simulink model "CranePIDv01"  (R2016b)
settings: Solver=ode45  StartTime=0.0  StopTime=280  RelTol=1e-3  EnableMultiTasking=on
PostLoadFcn:
  | plot_timeseries(Simulation_results);
undefined symbols (not defined in the file): A, adinchannels, adinchannelsencoders, adingain, adingainencoders, adinoffs, adinoffsencoders, B, C, D, daoutchannels, daoutgain, daoutoffs, h, Humusoft, MF634, sigbuilder_block
libraries: sldrtlib x3, simulink x3, dspsrcs4 x1
settings Model: Creator=rbabuska  LastModifiedBy=tcbooij
settings DataIOCC: LimitDataPoints=on  SaveFormat=Array
settings OptimizationCC: ExpressionDepthLimit=2147483647  LifeSpan=inf
settings DebuggingCC: AllowSymbolicDim=off  StateNameClashWarn=warning  SFUnexpectedBacktrackingDiag=warning  SFNoUnconditionalDefaultTransitionDiag=warning  SFExecutionAtInitializationDiag=none
settings HardwareCC: ProdBitPerPointer=32  ProdBitPerSizeT=32  ProdBitPerPtrDiffT=32  ProdLargestAtomicFloat=None  ProdIntDivRoundTo=Undefined  ProdEndianess=Unspecified  ProdWordSize=32  ProdHWDeviceType=32-bit Generic
settings ModelReferenceCC: PropagateSignalLabelsOutOfModel=off
settings GRTTargetCC: TargetLangStandard=C89/C90 (ANSI)  GeneratePreprocessorConditionals=Disable all  CombineOutputUpdateFcns=off  GRTInterface=on
settings ConfigComp: CovMetricSettings=dw  CovHtmlReporting=on  CovSaveCumulativeToWorkspaceVar=on  CovSaveSingleToWorkspaceVar=on  CovExternalEMLEnable=off

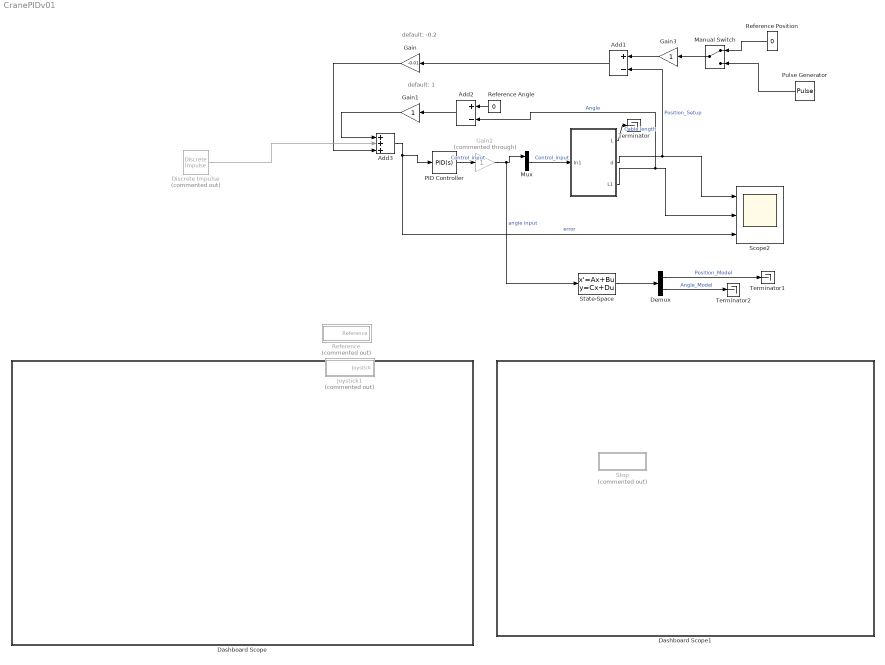
== system CranePIDv01 ==
  note: default: -0.2
  note: default: 1
  " Reference Angle" : Constant  Value=0
  " " : Subsystem  LoadFcn=hwinit  InitFcn=hwinit  mask{h=h}
      mask prompts: h "Sampling period [s]"
      mask Display: disp('Crane')
  Add1 : Sum  Inputs=+-
  Add2 : Sum  Inputs=+-
  Add3 : Sum  Inputs=3
  Dashboard Scope : Subsystem  DialogController=hmiCreateDDGDialog  IsWebBlock=on  mask(MWDashboardBlock){webBlockId=2a6f5fa7-1f9e-4fe4-9305-f01df55b8dfe, webBlockType=sdiscope, ShowInitialText=on, HMISrcModelName=CranePIDv01}
      mask prompts: webBlockId "WebBlock Id"; webBlockType "WebBlock Type"; HMISrcModelName "Source Model"
      mask help: SimulinkHMI:dialogs:HMIScopeDialogDesc
      mask Help: helpview([docroot '/mapfiles/simulink.map'], 'hmi_scope')
      mask Display:
      | if strcmp(get_param(bdroot(gcb),'BlockDiagramType'), 'library')
      |     image([(matlabroot) '/toolbox/simulink/hmi/icons/DashboardScope.png']);
      | end
  Dashboard Scope1 : Subsystem  DialogController=hmiCreateDDGDialog  IsWebBlock=on  mask(MWDashboardBlock){webBlockId=26260313-c547-41b7-b078-74ae54bbf42b, webBlockType=sdiscope, ShowInitialText=on, HMISrcModelName=CranePIDv01}
      mask prompts: webBlockId "WebBlock Id"; webBlockType "WebBlock Type"; HMISrcModelName "Source Model"
      mask help: SimulinkHMI:dialogs:HMIScopeDialogDesc
      mask Help: helpview([docroot '/mapfiles/simulink.map'], 'hmi_scope')
      mask Display:
      | if strcmp(get_param(bdroot(gcb),'BlockDiagramType'), 'library')
      |     image([(matlabroot) '/toolbox/simulink/hmi/icons/DashboardScope.png']);
      | end
  Demux : Demux  Outputs=2
  Discrete Impulse : dspsrcs4/Discrete  Impulse  Commented=on  Delay=0  SampleTime=1  FrameSample=1  OutputFrames=off  dataType=double  isSigned=on  wordLen=16  udDataType=sfix(16)  fracBitsMode=Best precision  numFracBits=15  OutDataTypeStr=double  LastOutDataTypeStr=double
  Gain : Gain  Gain=-0.01
  Gain1 : Gain
  Gain2 : Gain  Commented=through
  Gain3 : Gain
  Joystick1 : Subsystem  Commented=on
      mask Display: disp('Joystick')
  Manual Switch : ManualSwitch
  Mux : Mux  Inputs=2
  PID Controller : simulink/Continuous/PID Controller  Controller=PID  TimeDomain=Continuous-time  SampleTime=-1  IntegratorMethod=Forward Euler  FilterMethod=Forward Euler  Form=Parallel  UseFilter=on  ControllerParametersSource=internal  P=15  I=1  D=2  N=1  InitialConditionSource=internal  InitialConditionForIntegrator=0  InitialConditionForFilter=0  ExternalReset=none  LimitOutput=off  UpperSaturationLimit=inf  LowerSaturationLimit=-inf  LinearizeAsGain=on  AntiWindupMode=none  Kb=1  TrackingMode=off  Kt=1  PParamMin=[]  PParamMax=[]  IParamMin=[]  IParamMax=[]  DParamMin=[]  DParamMax=[]  NParamMin=[]  NParamMax=[]  KbParamMin=[]  KbParamMax=[]  KtParamMin=[]  KtParamMax=[]  POutMin=[]  POutMax=[]  IOutMin=[]  IOutMax=[]  DOutMin=[]  DOutMax=[]  NOutMin=[]  NOutMax=[]  KbOutMin=[]  KbOutMax=[]  KtOutMin=[]  KtOutMax=[]  IntegratorOutMin=[]  IntegratorOutMax=[]  FilterOutMin=[]  FilterOutMax=[]  SumOutMin=[]  SumOutMax=[]  SumI1OutMin=[]  SumI1OutMax=[]  SumI2OutMin=[]  SumI2OutMax=[]  SumI3OutMin=[]  SumI3OutMax=[]  SumDOutMin=[]  SumDOutMax=[]  SaturationOutMin=[]  SaturationOutMax=[]  IntegratorContinuousStateAttributes=''  IntegratorStateMustResolveToSignalObject=off  IntegratorRTWStateStorageClass=Auto  FilterContinuousStateAttributes=''  FilterStateMustResolveToSignalObject=off  FilterRTWStateStorageClass=Auto  DifferentiatorICPrevScaledInput=0  DifferentiatorOutMin=[]  DifferentiatorOutMax=[]
  Pulse Generator : DiscretePulseGenerator  PulseType=Time based  Amplitude=15  Period=20  PulseWidth=50  PhaseDelay=2
  Reference : Subsystem  Commented=on
      mask Display: disp('Reference')
  Reference Position : Constant  Value=0
  Scope2 : Scope  NumInputPorts=3
  State-Space : StateSpace  A=A  B=B  C=C  D=D  X0=0
  Stop : Subsystem  Commented=on
      mask Display: disp('Stop')
  Terminator : Terminator
  Terminator1 : Terminator
  Terminator2 : Terminator
  wires:
  " "/3(L1) -> Add2/2, Scope2/2  "Angle"
  " "/2(d) -> Add1/2, Scope2/1  "Position_Setup"
  Add3/1 -> PID Controller/1, Scope2/3  "error"
  " Reference Angle"/1 -> Add2/1
  Add2/1 -> Gain1/1
  Add1/1 -> Gain/1
  Gain/1 -> Add3/3
  Discrete Impulse/1 -> Add3/2
  Gain1/1 -> Add3/1
  " "/1(L) -> Terminator/1  "Cable length"
  PID Controller/1 -> Gain2/1  "Control_input"
  Mux/1 -> " "/1(In1)  "Control_input"
  Gain2/1 -> State-Space/1, Mux/1  "angle input"
  Gain3/1 -> Add1/1
  Reference Position/1 -> Manual Switch/1
  State-Space/1 -> Demux/1
  Demux/2 -> Terminator2/1  "Angle_Model"
  Demux/1 -> Terminator1/1  "Position_Model"
  Manual Switch/1 -> Gain3/1
  Pulse Generator/1 -> Manual Switch/2

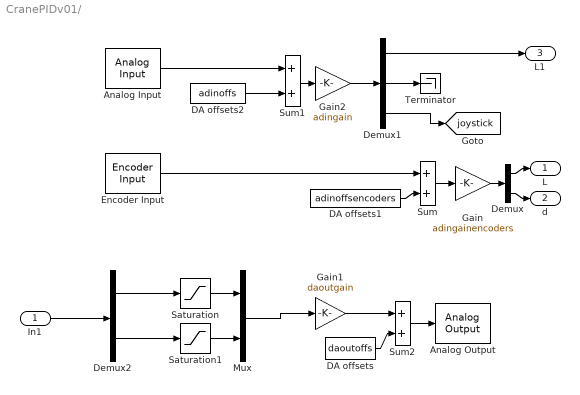
== system CranePIDv01/  ==
  In1 : Inport
  Analog Input : sldrtlib/Analog Input  SampleTime=h  MaxMissedTicks=ticklost  ShowMissedTicks=off  YieldWhenWaiting=off  DrvName=Humusoft/MF634  DrvAddress=4294967295  DrvOptions=0  Channels=[adinchannels]  RangeMode=2  VoltRange=1  DataType=1
      settings: AttributesFormatString=Humusoft\nMF634 [auto]
  Analog Output : sldrtlib/Analog Output  SampleTime=h  MaxMissedTicks=ticklost  ShowMissedTicks=off  YieldWhenWaiting=off  DrvName=Humusoft/MF634  DrvAddress=4294967295  DrvOptions=0  Channels=[daoutchannels]  RangeMode=2  VoltRange=1  InitialValue=0  FinalValue=0
      settings: AttributesFormatString=Humusoft\nMF634 [auto]
  DA offsets : Constant  Value=daoutoffs
  DA offsets1 : Constant  Value=adinoffsencoders
  DA offsets2 : Constant  Value=adinoffs
  Demux : Demux  Outputs=2
  Demux1 : Demux  Outputs=[1 1 2]
  Demux2 : Demux  Outputs=2
  Encoder Input : sldrtlib/Encoder Input  SampleTime=h  MaxMissedTicks=ticklost  ShowMissedTicks=off  YieldWhenWaiting=off  DrvName=Humusoft/MF634  DrvAddress=4294967295  DrvOptions=0  Channels=[adinchannelsencoders]  QuadMode=3  IndexPulse=1  InputFilter=Inf  DataType=1
      settings: AttributesFormatString=Humusoft\nMF634 [auto]
  Gain : Gain  Gain=adingainencoders  SaturateOnIntegerOverflow=on  OutDataTypeStr=Inherit: Same as input  ParamDataTypeStr=Inherit: Same as input
  Gain1 : Gain  Gain=daoutgain  SaturateOnIntegerOverflow=on  OutDataTypeStr=Inherit: Same as input  ParamDataTypeStr=Inherit: Same as input
  Gain2 : Gain  Gain=adingain  SaturateOnIntegerOverflow=on  OutDataTypeStr=Inherit: Same as input  ParamDataTypeStr=Inherit: Same as input
  Mux : Mux  Inputs=2
  Saturation : Saturate  UpperLimit=10  LowerLimit=-10
  Saturation1 : Saturate  UpperLimit=10  LowerLimit=-10
  Sum : Sum  SaturateOnIntegerOverflow=on  InputSameDT=on  OutDataTypeStr=Inherit: Same as first input
  Sum1 : Sum  SaturateOnIntegerOverflow=on  InputSameDT=on  OutDataTypeStr=Inherit: Same as first input
  Sum2 : Sum  SaturateOnIntegerOverflow=on  InputSameDT=on  OutDataTypeStr=Inherit: Same as first input
  Terminator : Terminator
  L : Outport  Tag=Position
  d : Outport  Tag=Cable length  Port=2
  L1 : Outport  Tag=Position  Port=3
  tag scope: joystick=global
  wires:
  Gain/1 -> Demux/1
  Sum/1 -> Gain/1
  DA offsets1/1 -> Sum/2
  Sum1/1 -> Gain2/1
  Analog Input/1 -> Sum1/1
  DA offsets2/1 -> Sum1/2
  Demux/1 -> L/1
  Demux/2 -> d/1
  Gain2/1 -> Demux1/1
  Demux1/3 -> [joystick]
  Demux1/1 -> L1/1
  Gain1/1 -> Sum2/1
  Sum2/1 -> Analog Output/1
  DA offsets/1 -> Sum2/2
  Encoder Input/1 -> Sum/1
  In1/1 -> Demux2/1
  Demux2/1 -> Saturation/1
  Demux2/2 -> Saturation1/1
  Saturation/1 -> Mux/1
  Mux/1 -> Gain1/1
  Saturation1/1 -> Mux/2
  Demux1/2 -> Terminator/1

== system CranePIDv01/Dashboard Scope ==

== system CranePIDv01/Dashboard Scope1 ==

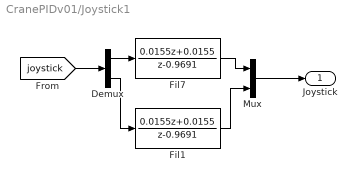
== system CranePIDv01/Joystick1 ==
  Demux : Demux  Outputs=2
  Fil1 : DiscreteTransferFcn  Numerator=[0.0155 0.0155]  Denominator=[1 -0.9691]  SampleTime=h
  Fil7 : DiscreteTransferFcn  Numerator=[0.0155 0.0155]  Denominator=[1 -0.9691]  SampleTime=h
  Mux : Mux  Inputs=2
  Joystick : Outport
  wires:
  Mux/1 -> Joystick/1
  Fil1/1 -> Mux/2
  Demux/2 -> Fil1/1
  Demux/1 -> Fil7/1
  [joystick] -> Demux/1
  Fil7/1 -> Mux/1

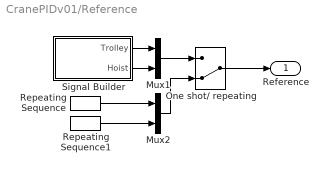
== system CranePIDv01/Reference ==
  Mux1 : Mux  Inputs=2
  Mux2 : Mux  Inputs=2
  One shot/ repeating : ManualSwitch  CurrentSetting=0
  Repeating Sequence : simulink/Sources/Repeating Sequence  rep_seq_t="[0    4.5000   12.5000   22.5000   30.5000   36.0000]"  rep_seq_y="[0         0    1.5000    1.5000         0         0]"
  Repeating Sequence1 : simulink/Sources/Repeating Sequence  rep_seq_t="[0     2     7    10    15    20    25    28    33    36]"  rep_seq_y="[0         0   -0.8000   -0.8000    0.3400    0.3400   -0.8000  -0.8000         0         0]"
  Signal Builder : Subsystem  Tag=STV Subsys  LoadFcn=sigbuilder_block('load');  StartFcn=sigbuilder_block('start');  StopFcn=sigbuilder_block('stop');  ClipboardFcn=sigbuilder_block('clipboard');  mask(Sigbuilder block){tuvar=[0:10]}
      mask help: Sigbuilder GUI
      mask init:
      | if ~strcmp(get_param(bdroot(gcb),'SimulationStatus'),'stopped') tuvar = sigbuilder_block('maskInit'); end
      settings: CopyFcn=sigbuilder_block('copy');  DeleteFcn=sigbuilder_block('delete');  ModelCloseFcn=sigbuilder_block('modelClose');  PreSaveFcn=sigbuilder_block('preSave');  PauseFcn=sigbuilder_block('pause')  ContinueFcn=sigbuilder_block('continue')  NameChangeFcn=sigbuilder_block('namechange');  OpenFcn=sigbuilder_block('open',[50.25 82.5 519.75 399.75 ]);  CloseFcn=sigbuilder_block('close');
      mask Display: plot(0,0,100,100,[10,10,40,40,10],[80,20,20,80,80],[40,10],[50,50], [40,27,10],[65,72,56],[40,25,25,10],[28,28,43,43]);
  Reference : Outport
  wires:
  Repeating Sequence1/1 -> Mux2/2
  Mux2/1 -> One shot/ repeating/2
  Repeating Sequence/1 -> Mux2/1
  Mux1/1 -> One shot/ repeating/1
  One shot/ repeating/1 -> Reference/1
  Signal Builder/1(Trolley) -> Mux1/1
  Signal Builder/2(Hoist) -> Mux1/2

== system CranePIDv01/Stop ==

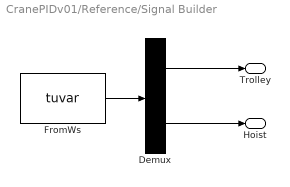
== system CranePIDv01/Reference/Signal Builder ==
  Demux : Demux  Tag=STV Demux  Outputs=2
  FromWs : FromWorkspace  Tag=STV FromWs  VariableName=tuvar  SampleTime=0
      SigBuilderData=|
      | dataSet.timeRange = [0 36]
      | dataSet.name = 'Group 1'
      | sbobj.Groups.Name = 'Group 1'
      | sbobj.Groups.Signals(1).Name = 'Trolley'
      | sbobj.Groups.Signals(1).XData = [0 4.5 12.5 22.5 30.5 36]
      | sbobj.Groups.Signals(1).YData = [0 0 1.5 1.5 0 0]
      | sbobj.Groups.Signals(2).Name = 'Hoist'
      | sbobj.Groups.Signals(2).XData = [0 2 7 10 15 20 25 28 33 36]
      | sbobj.Groups.Signals(2).YData = [0 0 -0.8 -0.8 0.34 0.34 -0.8 -0.8 0 0]
  Trolley : Outport  Tag=STV Outport
  Hoist : Outport  Tag=STV Outport  Port=2
  wires:
  Demux/2 -> Hoist/1
  Demux/1 -> Trolley/1
  FromWs/1 -> Demux/1
